simulink model "rx_20140509"  (R2012b)
settings: Solver=ode45  StartTime=0.0  StopTime=10000.0  RelTol=1e-3
libraries: xbsIndex_r4 x2065, casper_library_misc x67, xps_library x56, xbsReplacements_r4 x12, gavrt_library x3, casper_library_sources x2, simulink x1, casper_library_delays x1
(part 1 of 22)
settings Model: Creator=griffin  LastModifiedBy=wnew
settings DataIOCC: SignalLoggingSaveFormat=ModelDataLogs
settings DebuggingCC: FcnCallInpInsideContextMsg=UseLocalSettings  StrictBusMsg=Warning
settings GRTTargetCC: CombineOutputUpdateFcns=off  GRTInterface=on

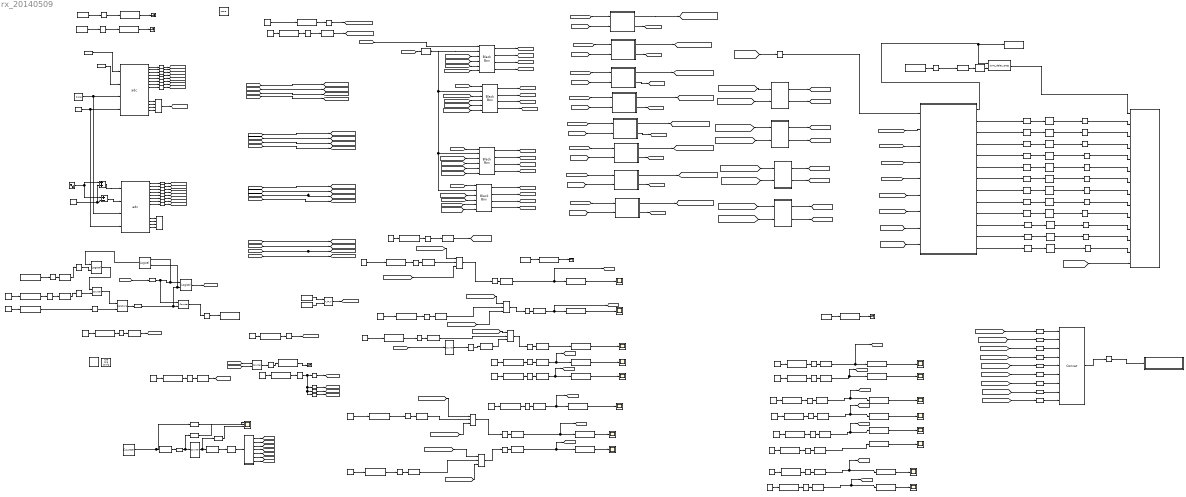
== system rx_20140509 ==
  note: fft_shift: bits 0-15
      | sync_rst: bit 16 -NA
      | arm_rst: bit 17 -NA
      | input_sel: bits 20-22
  note: The FFT Channels are assumed to be
      | Channel1= LCP +TREF (ADC0 I)
      | Channel2=LCP-TREF (ADC0 Q)
      | Channel3=RCP+TREF (ADC1 I)
      | Channel4=RCP-TREF (ADC1 Q)
  note: this shouild sync up the accumulation correctly
  note: To move DC bin higher:
      | Reduce Latency of Sync or increase latency of Data
      | To move DC bin lower:
      | Increase latency of Sync or decrease latency of Data
  note: 0 means Total Power/1 means Poalrimeter
  note: polarimeter versioning begins at 1
  " System Generator" : xbsIndex_r4/ System Generator  Tag=genX  xilinxfamily=virtex5  part=xc5vsx95t  speed=-1  package=ff1136  synthesis_tool=XST  clock_wrapper=Clock Enables  directory=./rx_20140505/sysgen  proj_type=Project Navigator  Synth_file=XST Defaults  Impl_file=ISE Defaults  testbench=off  simulink_period=1  sysclk_period=4  dcm_input_clock_period=100  incr_netlist=off  trim_vbits=Everywhere in SubSystem  dbl_ovrd=According to Block Masks  core_generation=According to Block Masks  run_coregen=off  deprecated_control=off  eval_field=0  block_type=sysgen
      settings: block_version=11.4
  Add2 : Sum
  Add3 : Sum  Inputs=+-
  Band-Limited White Noise1 : simulink/Sources/Band-Limited White Noise  Cov=0.000001  Ts=0.25  seed=[23341]
  Black Box{1..4} (4 alike) : xbsIndex_r4/Black Box  init_code=pfb_blackbox_200mhz_config  sim_method=Inactive  verbose=off  block_type=blackbox2
  Concat : xbsIndex_r4/Concat  num_inputs=9  dbl_ovrd=off  block_type=concat
  Constant{1,3..4,8} (4 alike) : Constant
  Constant{7,9..14,17..21,23..27} (17 alike) : Constant  Value=0
  Constant{2,5,15..16,22} (5 alike) : Constant  Value=30
  Convert : xbsIndex_r4/Convert  gui_display_data_type=Fixed-point  arith_type="Signed  (2's comp)"  n_bits=32  bin_pt=0  float_type=Single  exp_bits=8  fraction_bits=24  quantization=Truncate  overflow=Wrap  en=off  latency=0  dbl_ovrd=off  pipeline=off  block_type=convert
      settings: block_version=11.4
  Convert2 : xbsIndex_r4/Convert  gui_display_data_type=Fixed-point  arith_type=Boolean  n_bits=16  bin_pt=14  float_type=Single  exp_bits=8  fraction_bits=24  quantization=Truncate  overflow=Wrap  en=off  latency=0  dbl_ovrd=off  pipeline=off  block_type=convert
      settings: block_version=11.4
  Counter1 : xbsIndex_r4/Counter  cnt_type=Free Running  cnt_to=Inf  operation=Up  start_count=0  cnt_by_val=1  arith_type=Unsigned  n_bits=10  bin_pt=0  load_pin=off  rst=off  en=off  explicit_period=on  period=1  dbl_ovrd=off  use_behavioral_HDL=off  implementation=Fabric  block_type=counter
      settings: block_version=11.4
  Counter2 : xbsIndex_r4/Counter  cnt_type=Free Running  cnt_to=Inf  operation=Up  start_count=0  cnt_by_val=1  arith_type=Unsigned  n_bits=1  bin_pt=0  load_pin=off  rst=off  en=on  explicit_period=on  period=1  dbl_ovrd=off  use_behavioral_HDL=off  implementation=Fabric  block_type=counter
      settings: block_version=11.4
  Counter3 : xbsIndex_r4/Counter  cnt_type=Free Running  cnt_to=Inf  operation=Up  start_count=0  cnt_by_val=1  arith_type=Unsigned  n_bits=1  bin_pt=0  load_pin=off  rst=off  en=on  explicit_period=on  period=1  dbl_ovrd=off  use_behavioral_HDL=off  implementation=Fabric  block_type=counter
      settings: block_version=11.4
  Delay{,1,3,6,11..18,22,24..31,74..75,83,91} (25 alike) : xbsIndex_r4/Delay  rst=off  infoeditControl=Selection of Reset will increase slice count due to use of real FFs and instead of SRLs  en=off  latency=1  dbl_ovrd=off  reg_retiming=off  block_type=delay
      Delay11 settings: block_version=11.4
      Delay12 settings: block_version=11.4
      Delay13 settings: block_version=11.4
      Delay14 settings: block_version=11.4
      Delay15 settings: block_version=11.4
      Delay16 settings: block_version=11.4
      Delay17 settings: block_version=11.4
      Delay18 settings: block_version=11.4
      Delay22 settings: block_version=11.4
      Delay24 settings: block_version=11.4
      Delay25 settings: block_version=11.4
      Delay26 settings: block_version=11.4
      Delay27 settings: block_version=11.4
      Delay28 settings: block_version=11.4
      Delay29 settings: block_version=11.4
      Delay30 settings: block_version=11.4
  Delay{2,4..5,7..10,19..21,23,32..50,52,54..55,57..58,60,62,65,68,70,73,76..82,84..90,93..102} (65 alike) : xbsIndex_r4/Delay  rst=off  infoeditControl=Selection of Reset will increase slice count due to use of real FFs and instead of SRLs  en=off  latency=2  dbl_ovrd=off  reg_retiming=off  block_type=delay
  Delay{51,53,56,59,61,63..64,66..67,69,71..72} (12 alike) : xbsIndex_r4/Delay  rst=off  infoeditControl=Selection of Reset will increase slice count due to use of real FFs and instead of SRLs  en=off  latency=1  dbl_ovrd=off  reg_retiming=on  block_type=delay
  GPIOA_DIRECTION : xps_library/gpio  Tag=xps:gpio  io_group=ROACH:gpioa_oe_n  io_dir=out  arith_type=Boolean  bitwidth=1  bin_pt=0  bit_index=0  sample_period=1  use_single_ended=off  use_ddr=off  reg_iob=on  reg_clk_phase=0  termination=None
  GPIOB_DIRECTION : xps_library/gpio  Tag=xps:gpio  io_group=ROACH:gpiob_oe_n  io_dir=out  arith_type=Boolean  bitwidth=1  bin_pt=0  bit_index=0  sample_period=1  use_single_ended=off  use_ddr=off  reg_iob=on  reg_clk_phase=0  termination=None
  Imag : xbsIndex_r4/Constant  const=0  gui_display_data_type=Fixed-point  arith_type=Signed (2's comp)  n_bits=18  bin_pt=0  preci_type=Single  exp_width=8  frac_width=24  explicit_period=on  period=1  equ=P=C  opselect=C  inp2=PCIN>>17  opr=+  inp1=P  carry=CIN  dbl_ovrd=off  block_type=constant
      settings: block_version=11.4
  Logical : xbsIndex_r4/Logical  logical_function=OR  inputs=2  en=off  latency=2  precision=Full  arith_type=Unsigned  n_bits=16  bin_pt=0  align_bp=on  dbl_ovrd=off  block_type=logical
      settings: block_version=11.4
  Logical1 : xbsIndex_r4/Logical  logical_function=OR  inputs=4  en=off  latency=1  precision=Full  arith_type=Unsigned  n_bits=8  bin_pt=2  align_bp=on  dbl_ovrd=off  block_type=logical
      settings: xl_area=[1 1 0 1 0 0 0]
  Logical2 : xbsIndex_r4/Logical  logical_function=OR  inputs=2  en=off  latency=2  precision=Full  arith_type=Unsigned  n_bits=16  bin_pt=0  align_bp=on  dbl_ovrd=off  block_type=logical
      settings: block_version=11.4
  Logical3 : xbsIndex_r4/Logical  logical_function=OR  inputs=4  en=off  latency=1  precision=Full  arith_type=Unsigned  n_bits=8  bin_pt=2  align_bp=on  dbl_ovrd=off  block_type=logical
      settings: xl_area=[1 1 0 1 0 0 0]
  Logical4 : xbsIndex_r4/Logical  logical_function=OR  inputs=2  en=off  latency=2  precision=Full  arith_type=Unsigned  n_bits=16  bin_pt=0  align_bp=on  dbl_ovrd=off  block_type=logical
      settings: block_version=11.4
  Mux{,1..4} (5 alike) : xbsIndex_r4/Mux  inputs=2  en=off  latency=0  precision=Full  arith_type=Unsigned  n_bits=16  bin_pt=14  quantization=Truncate  overflow=Wrap  dbl_ovrd=off  block_type=mux
      settings: block_version=11.4
  Pulse Generator : DiscretePulseGenerator  Period=2^27
  Real : xbsIndex_r4/Constant  const=1  gui_display_data_type=Fixed-point  arith_type=Signed (2's comp)  n_bits=18  bin_pt=0  preci_type=Single  exp_width=8  frac_width=24  explicit_period=on  period=1  equ=P=C  opselect=C  inp2=PCIN>>17  opr=+  inp1=P  carry=CIN  dbl_ovrd=off  block_type=constant
      settings: block_version=11.4
  Real1 : xbsIndex_r4/Constant  const=0  gui_display_data_type=Fixed-point  arith_type=Boolean  n_bits=18  bin_pt=0  preci_type=Single  exp_width=8  frac_width=24  explicit_period=on  period=1  equ=P=C  opselect=C  inp2=PCIN>>17  opr=+  inp1=P  carry=CIN  dbl_ovrd=off  block_type=constant
      settings: block_version=11.4
  Real2 : xbsIndex_r4/Constant  const=0  gui_display_data_type=Fixed-point  arith_type=Boolean  n_bits=18  bin_pt=0  preci_type=Single  exp_width=8  frac_width=24  explicit_period=on  period=1  equ=P=C  opselect=C  inp2=PCIN>>17  opr=+  inp1=P  carry=CIN  dbl_ovrd=off  block_type=constant
      settings: block_version=11.4
  Real6 : xbsIndex_r4/Constant  const=1  gui_display_data_type=Fixed-point  arith_type=Unsigned  n_bits=18  bin_pt=0  preci_type=Single  exp_width=8  frac_width=24  explicit_period=on  period=1  equ=P=C  opselect=C  inp2=PCIN>>17  opr=+  inp1=P  carry=CIN  dbl_ovrd=off  block_type=constant
      settings: block_version=11.4
  Real7 : xbsIndex_r4/Constant  const=1  gui_display_data_type=Fixed-point  arith_type=Unsigned  n_bits=18  bin_pt=0  preci_type=Single  exp_width=8  frac_width=24  explicit_period=on  period=1  equ=P=C  opselect=C  inp2=PCIN>>17  opr=+  inp1=P  carry=CIN  dbl_ovrd=off  block_type=constant
      settings: block_version=11.4
  Reinterpret : xbsIndex_r4/Reinterpret  force_arith_type=on  arith_type=Unsigned  force_bin_pt=on  bin_pt=0  block_type=reinterpret
      settings: infoedit="Changes signal type without altering the binary representation.   You can changed the signal between signed and unsigned, and relocate the binary point.<br><br>Hardware notes: In hardware this block costs nothing.<br><br>Example:  Suppose the input is 6 bits wide, signed, with 2 fractional bits, and the output is forced to unsigned with 0 fractional bits.  Then an input of -2.0 (1110.00 in binary 2's complement) becomes an output of 56 (111000 in binary)."
  Relational : xbsIndex_r4/Relational  mode=a>b  en=off  latency=2  dbl_ovrd=off  block_type=relational
  Scope{,1..3,5..16} (16 alike) : Scope
      Scope settings: SaveName=ScopeData4
      Scope1 settings: SaveName=ScopeData10
      Scope10 settings: SaveName=ScopeData2
      Scope11 settings: YMin=0  YMax=1  SaveName=ScopeData3
      Scope12 settings: SaveName=ScopeData13
      Scope13 settings: SaveName=ScopeData14
      Scope14 settings: SaveName=ScopeData15
      Scope15 settings: SaveName=ScopeData16
      Scope16 settings: SaveName=ScopeData17
      Scope2 settings: YMin=0  YMax=1  SaveName=ScopeData11
      Scope5 settings: SaveName=ScopeData12
      Scope6 settings: SaveName=ScopeData7
      Scope7 settings: SaveName=ScopeData8
      Scope8 settings: SaveName=ScopeData9
      Scope9 settings: SaveName=ScopeData18
  Scope4 : Scope  NumInputPorts=3
      settings: YMin=-5~-5~-5  YMax=5~5~5
  Sine Wave1 : Sin  Amplitude=0.00001  Frequency=5  Phase=1.57  SampleTime=0.25
  Slice1 : xbsIndex_r4/Slice  nbits=1  boolean_output=on  mode=Upper Bit Location + Width  bit1=0  base1=LSB of Input  bit0=0  base0=LSB of Input  dbl_ovrd=off  block_type=slice
  Slice{5,9..17,21,23..36} (25 alike) : xbsIndex_r4/Slice  nbits=1  boolean_output=on  mode=Lower Bit Location + Width  bit1=0  base1=LSB of Input  bit0=0  base0=LSB of Input  dbl_ovrd=off  block_type=slice
  Slice18 : xbsIndex_r4/Slice  nbits=16  boolean_output=off  mode=Lower Bit Location + Width  bit1=0  base1=MSB of Input  bit0=0  base0=LSB of Input  dbl_ovrd=off  block_type=slice
      settings: infoedit="Extracts a given range of bits from each input sample and presents it at the output.  The output type is ordinarily unsigned with binary point at zero, but can be Boolean when the slice is one bit wide.<P><P>Hardware notes: In hardware this block costs nothing."  block_version=10.1.3
  Slice19 : xbsIndex_r4/Slice  nbits=1  boolean_output=on  mode=Lower Bit Location + Width  bit1=0  base1=MSB of Input  bit0=16  base0=LSB of Input  dbl_ovrd=off  block_type=slice
      settings: infoedit="Extracts a given range of bits from each input sample and presents it at the output.  The output type is ordinarily unsigned with binary point at zero, but can be Boolean when the slice is one bit wide.<P><P>Hardware notes: In hardware this block costs nothing."  block_version=10.1.3
  Slice2 : xbsIndex_r4/Slice  nbits=1  boolean_output=on  mode=Upper Bit Location + Width  bit1=0  base1=LSB of Input  bit0=0  base0=LSB of Input  dbl_ovrd=off  block_type=slice
  Slice20 : xbsIndex_r4/Slice  nbits=6  boolean_output=off  mode=Lower Bit Location + Width  bit1=0  base1=LSB of Input  bit0=0  base0=LSB of Input  dbl_ovrd=off  block_type=slice
  Slice22 : xbsIndex_r4/Slice  nbits=1  boolean_output=on  mode=Lower Bit Location + Width  bit1=0  base1=MSB of Input  bit0=17  base0=LSB of Input  dbl_ovrd=off  block_type=slice
      settings: infoedit="Extracts a given range of bits from each input sample and presents it at the output.  The output type is ordinarily unsigned with binary point at zero, but can be Boolean when the slice is one bit wide.<P><P>Hardware notes: In hardware this block costs nothing."  block_version=10.1.3
  Slice3 : xbsIndex_r4/Slice  nbits=3  boolean_output=off  mode=Lower Bit Location + Width  bit1=0  base1=MSB of Input  bit0=20  base0=LSB of Input  dbl_ovrd=off  block_type=slice
      settings: infoedit="Extracts a given range of bits from each input sample and presents it at the output.  The output type is ordinarily unsigned with binary point at zero, but can be Boolean when the slice is one bit wide.<P><P>Hardware notes: In hardware this block costs nothing."  block_version=10.1.3
  Slice4 : xbsIndex_r4/Slice  nbits=1  boolean_output=on  mode=Upper Bit Location + Width  bit1=0  base1=MSB of Input  bit0=0  base0=LSB of Input  dbl_ovrd=off  block_type=slice
  Slice7 : xbsIndex_r4/Slice  nbits=1  boolean_output=on  mode=Lower Bit Location + Width  bit1=-1  base1=MSB of Input  bit0=0  base0=LSB of Input  dbl_ovrd=off  block_type=slice
  Slice8 : xbsIndex_r4/Slice  nbits=1  boolean_output=on  mode=Lower Bit Location + Width  bit1=-1  base1=MSB of Input  bit0=0  base0=LSB of Input  dbl_ovrd=off  block_type=slice
  StokesDetector : Subsystem  AncestorBlock=gavrt_library/StokesDetector  mask(stokes){bit_width=18, add_latency=2, mult_latency=3}
      mask prompts: bit_width "Bit Width"; add_latency "Add Latency"; mult_latency "Mult Latency"
      mask help: Compute cross products necessary for full stokes parameters
  Subsystem1 : Subsystem
  Subsystem2 : Subsystem
  Subsystem3 : Subsystem
  Subsystem4 : Subsystem
  Subsystem5 : Subsystem
  Terminator{,1..4} (5 alike) : Terminator
  Walshing1 : Subsystem
  XSG core config : xps_library/XSG core config  Tag=xps:xsg  hw_sys=ROACH:sx95t  clk_src=adc0_clk  ROACH_clk_src=adc0_clk  ROACH2_clk_src=adc0_clk  clk_rate=250  sample_period=1  synthesis_tool=XST
  acc_len : xps_library/software register  Tag=xps:sw_reg  io_dir=From Processor  arith_type=Unsigned  bitwidth=32  bin_pt=0  sample_period=1  gw_name=rx_20140509_acc_len_user_data_out
  acc_sync_delay : xps_library/software register  Tag=xps:sw_reg  io_dir=From Processor  arith_type=Unsigned  bitwidth=32  bin_pt=0  sample_period=1  gw_name=rx_20140509_acc_sync_delay_user_data_out
  adc0 : xps_library/adc  Tag=xps:adc  adc_brd=adc0  adc_clk_rate=1000  adc_interleave=off  sample_period=1
  adc1 : xps_library/adc  Tag=xps:adc  adc_brd=adc1  adc_clk_rate=1000  adc_interleave=off  sample_period=1
  amp_EQ0 : Subsystem  mask{N=5, bram_lat=2, mult_lat=3, add_lat=2}
      mask prompts: N "number of coefficients (2^?)"; bram_lat "bram latency"; mult_lat "multiplier latency"; add_lat "adder latency"
  amp_EQ1 : Subsystem  mask{N=5, bram_lat=2, mult_lat=3, add_lat=2}
      mask prompts: N "number of coefficients (2^?)"; bram_lat "bram latency"; mult_lat "multiplier latency"; add_lat "adder latency"
  amp_EQ2 : Subsystem  mask{N=5, bram_lat=2, mult_lat=3, add_lat=2}
      mask prompts: N "number of coefficients (2^?)"; bram_lat "bram latency"; mult_lat "multiplier latency"; add_lat "adder latency"
  amp_EQ3 : Subsystem  mask{N=5, bram_lat=2, mult_lat=3, add_lat=2}
      mask prompts: N "number of coefficients (2^?)"; bram_lat "bram latency"; mult_lat "multiplier latency"; add_lat "adder latency"
  amp_EQ4 : Subsystem  mask{N=5, bram_lat=2, mult_lat=3, add_lat=2}
      mask prompts: N "number of coefficients (2^?)"; bram_lat "bram latency"; mult_lat "multiplier latency"; add_lat "adder latency"
  amp_EQ5 : Subsystem  mask{N=5, bram_lat=2, mult_lat=3, add_lat=2}
      mask prompts: N "number of coefficients (2^?)"; bram_lat "bram latency"; mult_lat "multiplier latency"; add_lat "adder latency"
  amp_EQ6 : Subsystem  mask{N=5, bram_lat=2, mult_lat=3, add_lat=2}
      mask prompts: N "number of coefficients (2^?)"; bram_lat "bram latency"; mult_lat "multiplier latency"; add_lat "adder latency"
  amp_EQ7 : Subsystem  mask{N=5, bram_lat=2, mult_lat=3, add_lat=2}
      mask prompts: N "number of coefficients (2^?)"; bram_lat "bram latency"; mult_lat "multiplier latency"; add_lat "adder latency"
  bofMode : xps_library/software register  Tag=xps:sw_reg  io_dir=From Processor  arith_type=Unsigned  bitwidth=32  bin_pt=0  sample_period=1  gw_name=rx_20140509_bofMode_user_data_out
  bofVersion : xps_library/software register  Tag=xps:sw_reg  io_dir=From Processor  arith_type=Unsigned  bitwidth=32  bin_pt=0  sample_period=1  gw_name=rx_20140509_bofVersion_user_data_out
  cnt_rst : xps_library/software register  Tag=xps:sw_reg  io_dir=From Processor  arith_type=Unsigned  bitwidth=32  bin_pt=0  sample_period=1  gw_name=rx_20140509_cnt_rst_user_data_out
  ctrl_sw : xps_library/software register  Tag=xps:sw_reg  io_dir=From Processor  arith_type=Unsigned  bitwidth=32  bin_pt=0  sample_period=1  gw_name=rx_20140509_ctrl_sw_user_data_out
  demodPhaseSwitch1 : xps_library/software register  Tag=xps:sw_reg  io_dir=From Processor  arith_type=Unsigned  bitwidth=32  bin_pt=0  sample_period=1  gw_name=rx_20140509_demodPhaseSwitch1_user_data_out
  gpio : xps_library/gpio  Tag=xps:gpio  io_group=ROACH:gpioa  io_dir=out  arith_type=Boolean  bitwidth=1  bin_pt=0  bit_index=0  sample_period=1  use_single_ended=off  use_ddr=off  reg_iob=on  reg_clk_phase=0  termination=None
  gpio1 : xps_library/gpio  Tag=xps:gpio  io_group=ROACH:gpioa  io_dir=out  arith_type=Boolean  bitwidth=1  bin_pt=0  bit_index=1  sample_period=1  use_single_ended=off  use_ddr=off  reg_iob=on  reg_clk_phase=0  termination=None
  gpio10 : xps_library/gpio  Tag=xps:gpio  io_group=ROACH:gpiob  io_dir=out  arith_type=Boolean  bitwidth=1  bin_pt=0  bit_index=2  sample_period=1  use_single_ended=off  use_ddr=off  reg_iob=on  reg_clk_phase=0  termination=None
  gpio11 : xps_library/gpio  Tag=xps:gpio  io_group=ROACH:gpiob  io_dir=out  arith_type=Boolean  bitwidth=1  bin_pt=0  bit_index=3  sample_period=1  use_single_ended=off  use_ddr=off  reg_iob=on  reg_clk_phase=0  termination=None
  gpio12 : xps_library/gpio  Tag=xps:gpio  io_group=ROACH:gpiob  io_dir=out  arith_type=Boolean  bitwidth=1  bin_pt=0  bit_index=4  sample_period=1  use_single_ended=off  use_ddr=off  reg_iob=on  reg_clk_phase=0  termination=None
  gpio13 : xps_library/gpio  Tag=xps:gpio  io_group=ROACH:gpiob  io_dir=out  arith_type=Boolean  bitwidth=1  bin_pt=0  bit_index=5  sample_period=1  use_single_ended=off  use_ddr=off  reg_iob=on  reg_clk_phase=0  termination=None
  gpio14 : xps_library/gpio  Tag=xps:gpio  io_group=ROACH:gpiob  io_dir=out  arith_type=Boolean  bitwidth=1  bin_pt=0  bit_index=6  sample_period=1  use_single_ended=off  use_ddr=off  reg_iob=on  reg_clk_phase=0  termination=None
  gpio15 : xps_library/gpio  Tag=xps:gpio  io_group=ROACH:gpiob  io_dir=out  arith_type=Boolean  bitwidth=1  bin_pt=0  bit_index=7  sample_period=1  use_single_ended=off  use_ddr=off  reg_iob=on  reg_clk_phase=0  termination=None
  gpio2 : xps_library/gpio  Tag=xps:gpio  io_group=ROACH:gpioa  io_dir=out  arith_type=Boolean  bitwidth=1  bin_pt=0  bit_index=2  sample_period=1  use_single_ended=off  use_ddr=off  reg_iob=on  reg_clk_phase=0  termination=None
  gpio3 : xps_library/gpio  Tag=xps:gpio  io_group=ROACH:gpioa  io_dir=out  arith_type=Boolean  bitwidth=1  bin_pt=0  bit_index=3  sample_period=1  use_single_ended=off  use_ddr=off  reg_iob=on  reg_clk_phase=0  termination=None
  gpio4 : xps_library/gpio  Tag=xps:gpio  io_group=ROACH:gpioa  io_dir=out  arith_type=Boolean  bitwidth=1  bin_pt=0  bit_index=4  sample_period=1  use_single_ended=off  use_ddr=off  reg_iob=on  reg_clk_phase=0  termination=None
  gpio5 : xps_library/gpio  Tag=xps:gpio  io_group=ROACH:gpioa  io_dir=out  arith_type=Boolean  bitwidth=1  bin_pt=0  bit_index=5  sample_period=1  use_single_ended=off  use_ddr=off  reg_iob=on  reg_clk_phase=0  termination=None
  gpio6 : xps_library/gpio  Tag=xps:gpio  io_group=ROACH:gpioa  io_dir=out  arith_type=Boolean  bitwidth=1  bin_pt=0  bit_index=6  sample_period=1  use_single_ended=off  use_ddr=off  reg_iob=on  reg_clk_phase=0  termination=None
  gpio7 : xps_library/gpio  Tag=xps:gpio  io_group=ROACH:gpioa  io_dir=out  arith_type=Boolean  bitwidth=1  bin_pt=0  bit_index=7  sample_period=1  use_single_ended=off  use_ddr=off  reg_iob=on  reg_clk_phase=0  termination=None
  gpio8 : xps_library/gpio  Tag=xps:gpio  io_group=ROACH:gpiob  io_dir=out  arith_type=Boolean  bitwidth=1  bin_pt=0  bit_index=0  sample_period=1  use_single_ended=off  use_ddr=off  reg_iob=on  reg_clk_phase=0  termination=None
  gpio9 : xps_library/gpio  Tag=xps:gpio  io_group=ROACH:gpiob  io_dir=out  arith_type=Boolean  bitwidth=1  bin_pt=0  bit_index=1  sample_period=1  use_single_ended=off  use_ddr=off  reg_iob=on  reg_clk_phase=0  termination=None
  gpioMode : xps_library/software register  Tag=xps:sw_reg  io_dir=From Processor  arith_type=Unsigned  bitwidth=32  bin_pt=0  sample_period=1  gw_name=rx_20140509_gpioMode_user_data_out
  gpio_set0 : xps_library/software register  Tag=xps:sw_reg  io_dir=From Processor  arith_type=Unsigned  bitwidth=32  bin_pt=0  sample_period=1  gw_name=rx_20140509_gpio_set0_user_data_out
  gpio_set1 : xps_library/software register  Tag=xps:sw_reg  io_dir=From Processor  arith_type=Unsigned  bitwidth=32  bin_pt=0  sample_period=1  gw_name=rx_20140509_gpio_set1_user_data_out
  gpio_set2 : xps_library/software register  Tag=xps:sw_reg  io_dir=From Processor  arith_type=Unsigned  bitwidth=32  bin_pt=0  sample_period=1  gw_name=rx_20140509_gpio_set2_user_data_out
  gpio_set3 : xps_library/software register  Tag=xps:sw_reg  io_dir=From Processor  arith_type=Unsigned  bitwidth=32  bin_pt=0  sample_period=1  gw_name=rx_20140509_gpio_set3_user_data_out
  gpio_set4 : xps_library/software register  Tag=xps:sw_reg  io_dir=From Processor  arith_type=Unsigned  bitwidth=32  bin_pt=0  sample_period=1  gw_name=rx_20140509_gpio_set4_user_data_out
  gpio_set5 : xps_library/software register  Tag=xps:sw_reg  io_dir=From Processor  arith_type=Unsigned  bitwidth=32  bin_pt=0  sample_period=1  gw_name=rx_20140509_gpio_set5_user_data_out
  gpio_set6 : xps_library/software register  Tag=xps:sw_reg  io_dir=From Processor  arith_type=Unsigned  bitwidth=32  bin_pt=0  sample_period=1  gw_name=rx_20140509_gpio_set6_user_data_out
  gpio_set7 : xps_library/software register  Tag=xps:sw_reg  io_dir=From Processor  arith_type=Unsigned  bitwidth=32  bin_pt=0  sample_period=1  gw_name=rx_20140509_gpio_set7_user_data_out
  gpiob_set0 : xps_library/software register  Tag=xps:sw_reg  io_dir=From Processor  arith_type=Unsigned  bitwidth=32  bin_pt=0  sample_period=1  gw_name=rx_20140509_gpiob_set0_user_data_out
  gpiob_set1 : xps_library/software register  Tag=xps:sw_reg  io_dir=From Processor  arith_type=Unsigned  bitwidth=32  bin_pt=0  sample_period=1  gw_name=rx_20140509_gpiob_set1_user_data_out
  gpiob_set2 : xps_library/software register  Tag=xps:sw_reg  io_dir=From Processor  arith_type=Unsigned  bitwidth=32  bin_pt=0  sample_period=1  gw_name=rx_20140509_gpiob_set2_user_data_out
  gpiob_set3 : xps_library/software register  Tag=xps:sw_reg  io_dir=From Processor  arith_type=Unsigned  bitwidth=32  bin_pt=0  sample_period=1  gw_name=rx_20140509_gpiob_set3_user_data_out
  gpiob_set4 : xps_library/software register  Tag=xps:sw_reg  io_dir=From Processor  arith_type=Unsigned  bitwidth=32  bin_pt=0  sample_period=1  gw_name=rx_20140509_gpiob_set4_user_data_out
  gpiob_set5 : xps_library/software register  Tag=xps:sw_reg  io_dir=From Processor  arith_type=Unsigned  bitwidth=32  bin_pt=0  sample_period=1  gw_name=rx_20140509_gpiob_set5_user_data_out
  gpiob_set6 : xps_library/software register  Tag=xps:sw_reg  io_dir=From Processor  arith_type=Unsigned  bitwidth=32  bin_pt=0  sample_period=1  gw_name=rx_20140509_gpiob_set6_user_data_out
  gpiob_set7 : xps_library/software register  Tag=xps:sw_reg  io_dir=From Processor  arith_type=Unsigned  bitwidth=32  bin_pt=0  sample_period=1  gw_name=rx_20140509_gpiob_set7_user_data_out
  no_PPS_cnt : xps_library/software register  Tag=xps:sw_reg  io_dir=To Processor  arith_type=Unsigned  bitwidth=32  bin_pt=0  sample_period=1  gw_name=rx_20140509_no_PPS_cnt_user_data_in
  out : xbsIndex_r4/Gateway Out  inherit_from_input=off  hdl_port=on  timing_constraint=None  locs_specified=off  LOCs={}  UseAsDAC=off  DACChannel='1'  block_type=gatewayout
      settings: infoedit="Gateway out block.  Converts Xilinx fixed point inputs into ouputs of type Simulink integer, double, or fixed point.<br><br>Hardware notes:  In hardware these blocks become top level output ports or are discarded, depending on how they are configured."  block_version=11.4
  out1 : xbsIndex_r4/Gateway Out  inherit_from_input=off  hdl_port=on  timing_constraint=None  locs_specified=off  LOCs={}  UseAsDAC=off  DACChannel='1'  block_type=gatewayout
      settings: infoedit="Gateway out block.  Converts Xilinx fixed point inputs into ouputs of type Simulink integer, double, or fixed point.<br><br>Hardware notes:  In hardware these blocks become top level output ports or are discarded, depending on how they are configured."  block_version=11.4
  out2 : xbsIndex_r4/Gateway Out  inherit_from_input=off  hdl_port=on  timing_constraint=None  locs_specified=off  LOCs={}  UseAsDAC=off  DACChannel='1'  block_type=gatewayout
      settings: infoedit="Gateway out block.  Converts Xilinx fixed point inputs into ouputs of type Simulink integer, double, or fixed point.<br><br>Hardware notes:  In hardware these blocks become top level output ports or are discarded, depending on how they are configured."  block_version=11.4
  pcore : xps_library/pcore  Tag=xps:pcore  pcore_path=./pfb_blackbox_200mhz_core/pfb_blackbox_200mhz.ngc
  phaseDelay2 : xps_library/software register  Tag=xps:sw_reg  io_dir=From Processor  arith_type=Unsigned  bitwidth=32  bin_pt=0  sample_period=1  gw_name=rx_20140509_phaseDelay2_user_data_out
  posedge1 : casper_library_misc/posedge  Tag=Rising Edge Detector
  posedge2 : casper_library_misc/posedge  Tag=Rising Edge Detector
  posedge6 : casper_library_misc/posedge  Tag=Rising Edge Detector
  pure_tone_gen : casper_library_sources/pure_tone_gen  adc_demux_factor=8  num_fft_channels=32  tone_channel=10
  pure_tone_gen1 : casper_library_sources/pure_tone_gen  adc_demux_factor=8  num_fft_channels=32  tone_channel=10
  ri_to_c8 : casper_library_misc/ri_to_c
  snap_we : xps_library/software register  Tag=xps:sw_reg  io_dir=From Processor  arith_type=Unsigned  bitwidth=32  bin_pt=0  sample_period=1  gw_name=rx_20140509_snap_we_user_data_out
  statusReadout : Subsystem  Tag=xps:sw_reg  mask{io_dir=To Processor, arith_type=Unsigned, bitwidth=32, bin_pt=0, sample_period=1, latency=0}
      mask prompts: io_dir "I/O direction"; arith_type "Data Type"; bitwidth "Data bitwidth"; bin_pt "Data binary point"; sample_period "Sample period"
      mask init:
      | gw_name = clear_name(gcb);
      | config.source = str2func('software_register_init');
      | config.toplevel = gcb;
      | xBlock( config, {io_dir, arith_type, bitwidth, bin_pt, ... 
      |     sample_period, gw_name, latency});
      mask TypeOptions io_dir: From Processor | To Processor
      mask TypeOptions arith_type: Unsigned | Signed  (2's comp)
  sync : xbsIndex_r4/Counter  cnt_type=Free Running  cnt_to=Inf  operation=Up  start_count=0  cnt_by_val=1  arith_type=Unsigned  n_bits=29  bin_pt=0  load_pin=off  rst=on  en=on  explicit_period=on  period=1  dbl_ovrd=off  use_behavioral_HDL=off  implementation=Fabric  block_type=counter
      settings: block_version=11.4
  sync1 : xbsIndex_r4/Counter  cnt_type=Free Running  cnt_to=Inf  operation=Up  start_count=0  cnt_by_val=1  arith_type=Unsigned  n_bits=29  bin_pt=0  load_pin=off  rst=on  en=on  explicit_period=on  period=1  dbl_ovrd=off  use_behavioral_HDL=off  implementation=Fabric  block_type=counter
      settings: block_version=11.4
  sync_cnt : xps_library/software register  Tag=xps:sw_reg  io_dir=To Processor  arith_type=Unsigned  bitwidth=32  bin_pt=0  sample_period=1  gw_name=rx_20140509_sync_cnt_user_data_in
  sync_cnt1 : xps_library/software register  Tag=xps:sw_reg  io_dir=To Processor  arith_type=Unsigned  bitwidth=32  bin_pt=0  sample_period=1  gw_name=rx_20140509_sync_cnt1_user_data_in
  sync_cntr : xbsIndex_r4/Counter  cnt_type=Free Running  cnt_to=Inf  operation=Up  start_count=0  cnt_by_val=1  arith_type=Unsigned  n_bits=32  bin_pt=0  load_pin=off  rst=on  en=on  explicit_period=on  period=1  dbl_ovrd=off  use_behavioral_HDL=off  implementation=Fabric  block_type=counter
      settings: block_version=11.4
  sync_delay_prog : casper_library_delays/sync_delay_prog  MaxDelay=6
  sync_en : xps_library/software register  Tag=xps:sw_reg  io_dir=From Processor  arith_type=Unsigned  bitwidth=32  bin_pt=0  sample_period=1  gw_name=rx_20140509_sync_en_user_data_out
  sync_max : xps_library/software register  Tag=xps:sw_reg  io_dir=From Processor  arith_type=Unsigned  bitwidth=32  bin_pt=0  sample_period=1  gw_name=rx_20140509_sync_max_user_data_out
  sync_rst : xps_library/software register  Tag=xps:sw_reg  io_dir=From Processor  arith_type=Unsigned  bitwidth=32  bin_pt=0  sample_period=1  gw_name=rx_20140509_sync_rst_user_data_out
      link override rx_25May_stat_sync_rst_user_data_out: gui_display_data_type=Boolean  arith_type=Boolean  n_bits=32  bin_pt=0  preci_type=Single  exp_width=8  frac_width=24  quantization="Round  (unbiased: +/- Inf)"  overflow=Saturate  period=1  dbl_ovrd=off  timing_constraint=None  locs_specified=off  LOCs={}  UseAsADC=off  ADCChannel='1'  inherit_from_input=off  hdl_port=on
      link override rx_25May_stat_sync_rst_user_data_out: infoedit="Gateway in block.  Converts inputs of type Simulink integer, single, double and fixed-point to  Xilinx fixed-point or floating-point data type.<br><br>Hardware notes:  In hardware these blocks become top level input ports."
  wires:
  Slice22/1 -> [arm_rst]
  Slice19/1 -> [sync_rst]
  Slice18/1 -> [fft_shift]
  Slice3/1 -> [input_sel]
  Delay/1 -> Slice3/1, Slice22/1, Slice19/1, Slice18/1
  ctrl_sw/1 -> Delay/1
  Constant18/1 -> ctrl_sw/1
  Imag/1 -> ri_to_c8/2
  ri_to_c8/1 -> [unity]
  Real/1 -> ri_to_c8/1
  acc_len/1 -> Delay1/1
  Constant2/1 -> acc_len/1
  Delay1/1 -> [acc_len]
  Delay2/1 -> sync_cnt/1
  sync_cntr/1 -> Delay2/1
  sync_cnt/1 -> Terminator/1
  [sync_gen] -> sync_cntr/2
  cnt_rst/1 -> Delay4/1
  Delay4/1 -> Slice1/1
  Slice1/1 -> [cnt_rst]
  Constant3/1 -> cnt_rst/1
  [cnt_rst] -> sync_cntr/1
  Pulse Generator/1 -> adc0/3, adc1/3
  Constant1/1 -> adc0/4, adc1/4
  adc0/13 -> Logical3/1
  adc0/14 -> Logical3/2
  adc0/15 -> Logical3/3
  adc0/16 -> Logical3/4
  adc0/1 -> Delay22/1
  adc0/2 -> Delay24/1
  adc0/3 -> Delay25/1
  adc0/4 -> Delay26/1
  adc0/5 -> Delay27/1
  adc0/6 -> Delay28/1
  adc0/7 -> Delay29/1
  adc0/8 -> Delay30/1
  Logical3/1 -> [sync_adc0]
  Delay22/1 -> [adc0_lcp0]
  Delay24/1 -> [adc0_lcp1]
  Delay25/1 -> [adc0_lcp2]
  Delay26/1 -> [adc0_lcp3]
  Delay27/1 -> [adc0_lcp0a]
  Delay28/1 -> [adc0_lcp1a]
  Delay29/1 -> [adc0_lcp2a]
  Delay30/1 -> [adc0_lcp3a]
  adc1/13 -> Logical1/1
  adc1/14 -> Logical1/2
  adc1/15 -> Logical1/3
  adc1/16 -> Logical1/4
  adc1/1 -> Delay11/1
  adc1/2 -> Delay12/1
  adc1/3 -> Delay13/1
  adc1/4 -> Delay14/1
  adc1/5 -> Delay15/1
  adc1/6 -> Delay16/1
  adc1/7 -> Delay17/1
  adc1/8 -> Delay18/1
  Delay11/1 -> [adc0_rcp0]
  Delay12/1 -> [adc0_rcp1]
  Delay13/1 -> [adc0_rcp2]
  Delay14/1 -> [adc0_rcp3]
  Delay15/1 -> [adc0_rcp0a]
  Delay16/1 -> [adc0_rcp1a]
  Delay17/1 -> [adc0_rcp2a]
  Delay18/1 -> [adc0_rcp3a]
  pure_tone_gen/1 -> adc0/1
  pure_tone_gen1/1 -> adc0/2
  Add2/1 -> adc1/1
  Add3/1 -> adc1/2
  Band-Limited White Noise1/1 -> Add3/2, Add2/2
  Sine Wave1/1 -> Add2/1, Add3/1
  snap_we/1 -> Delay5/1
  Delay5/1 -> Slice2/1
  Slice2/1 -> [snap_we]
  Constant4/1 -> snap_we/1
  [sync_gen] -> Black Box3/1
  [adc0_lcp3demod] -> Black Box3/6
  [adc0_lcp0demod] -> Black Box3/3
  [adc0_lcp1demod] -> Black Box3/4
  [adc0_lcp2demod] -> Black Box3/5
  Black Box3/1 -> [fft0_sync]
  Black Box3/2 -> [fft0_lcp_even]
  Black Box3/3 -> [fft0_lcp_odd]
  Black Box3/4 -> [fft0_of]
  [sync_gen] -> Black Box1/1
  [adc0_lcp0ademod] -> Black Box1/3
  [adc0_lcp1ademod] -> Black Box1/4
  [adc0_lcp2ademod] -> Black Box1/5
  [adc0_lcp3ademod] -> Black Box1/6
  Black Box1/1 -> [fft1_sync]
  Black Box1/2 -> [fft1_lcp_even]
  Black Box1/3 -> [fft1_lcp_odd]
  Black Box1/4 -> [fft1_of]
  [sync_gen] -> Black Box2/1
  [adc0_rcp0ademod] -> Black Box2/3
  [adc0_rcp1ademod] -> Black Box2/4
  [adc0_rcp2ademod] -> Black Box2/5
  [adc0_rcp3ademod] -> Black Box2/6
  [sync_gen] -> Black Box4/1
  [adc0_rcp0demod] -> Black Box4/3
  [adc0_rcp1demod] -> Black Box4/4
  [adc0_rcp2demod] -> Black Box4/5
  [adc0_rcp3demod] -> Black Box4/6
  Black Box4/1 -> [fft2_sync]
  Black Box4/2 -> [fft2_rcp_even]
  Black Box4/3 -> [fft2_rcp_odd]
  Black Box4/4 -> [fft2_of]
  Black Box2/1 -> [fft3_sync]
  Black Box2/2 -> [fft3_rcp_even]
  Black Box2/3 -> [fft3_rcp_odd]
  Black Box2/4 -> [fft3_of]
  [fft_shift] -> Convert/1
  Convert/1 -> Black Box3/2, Black Box1/2, Black Box2/2, Black Box4/2
  Real1/1 -> GPIOA_DIRECTION/1
  GPIOA_DIRECTION/1 -> Terminator3/1
  [fft0_sync] -> amp_EQ1/1(sync_in)
  [fft0_lcp_odd] -> amp_EQ1/2(din)
  [fft0_lcp_even] -> amp_EQ0/2(din)
  [fft0_sync] -> amp_EQ0/1(sync_in)
  [fft1_sync] -> amp_EQ3/1(sync_in)
  [fft1_lcp_odd] -> amp_EQ3/2(din)
  [fft1_sync] -> amp_EQ2/1(sync_in)
  [fft1_lcp_even] -> amp_EQ2/2(din)
  [fft2_sync] -> amp_EQ5/1(sync_in)
  [fft2_rcp_odd] -> amp_EQ5/2(din)
  [fft2_sync] -> amp_EQ4/1(sync_in)
  [fft2_rcp_even] -> amp_EQ4/2(din)
  [fft3_sync] -> amp_EQ7/1(sync_in)
  [fft3_rcp_odd] -> amp_EQ7/2(din)
  [fft3_sync] -> amp_EQ6/1(sync_in)
  [fft3_rcp_even] -> amp_EQ6/2(din)
  Walshing1/1(Out1) -> [wal0]
  Walshing1/2(Out2) -> [wal1]
  Walshing1/3(Out3) -> [wal2]
  Walshing1/4(Out4) -> [wal3]
  Walshing1/5(Out5) -> [wal4]
  Walshing1/6(Out6) -> [wal5]
  Walshing1/7(Out7) -> [wal6]
  Counter1/1 -> out/1, Slice4/1
  Counter3/1 -> Slice10/1, out2/1
  Slice10/1 -> Convert2/1
  Convert2/1 -> Walshing1/1(CLK)
  out/1 -> Scope4/1
  out1/1 -> Scope4/2
  out2/1 -> Scope4/3
  posedge2/1 -> Counter3/1, out1/1
  Slice4/1 -> posedge2/1
  gpio2/1 -> Scope2/1
  Slice9/1 -> gpio2/1
  Delay20/1 -> Slice9/1
  gpio_set3/1 -> Delay19/1
  Constant9/1 -> gpio_set3/1
  gpio3/1 -> Scope3/1
  Slice5/1 -> gpio3/1, [gpioa3]
  Delay19/1 -> Slice5/1
  Delay41/1 -> Slice11/1
  Delay47/1 -> Slice12/1
  gpio_set5/1 -> Delay23/1
  Constant8/1 -> gpio_set5/1
  gpio5/1 -> Scope5/1
  Slice14/1 -> gpio5/1, [gpioa5]
  Delay23/1 -> Slice14/1
  gpio_set4/1 -> Delay21/1
  Constant10/1 -> gpio_set4/1
  gpio4/1 -> Scope6/1
  Slice13/1 -> gpio4/1, [gpioa4]
  Delay21/1 -> Slice13/1
  Delay45/1 -> Slice15/1
  Delay46/1 -> Slice16/1
  Slice11/1 -> [wal0gpio], gpio6/1
  Slice12/1 -> [wal1gpio], gpio7/1
  gpio7/1 -> Scope1/1
  gpio6/1 -> Scope/1
  gpio/1 -> Scope7/1
  Slice16/1 -> gpio1/1, [wal3gpio]
  gpio1/1 -> Scope8/1
  [sync_gen] -> Counter2/1
  acc_sync_delay/1 -> Delay6/1
  Delay6/1 -> Slice20/1
  Slice20/1 -> Reinterpret/1
  Reinterpret/1 -> sync_delay_prog/2
  Delay64/1 -> Delay57/1
  Delay59/1 -> Delay58/1
  Delay61/1 -> Delay60/1
  Delay63/1 -> Delay62/1
  demodPhaseSwitch1/1 -> Delay3/1
  Constant15/1 -> demodPhaseSwitch1/1
  Delay3/1 -> Slice21/1
  Slice21/1 -> [demodPhaseSwitch]
  Constant16/1 -> phaseDelay2/1
  phaseDelay2/1 -> Delay31/1
  Delay31/1 -> [phaseDelay1]
  Delay57/1 -> Delay40/1
  Delay58/1 -> Delay42/1
  Delay60/1 -> Delay43/1
  Delay62/1 -> Delay44/1
  [Vsky_Add_Vload_LCP_Odd] -> Subsystem3/1(In1)
  [Vsky_Sub_Vload_LCP_Odd] -> Subsystem3/2(In2)
  [Vsky_Add_Vload_LCP_Even] -> Subsystem5/1(In1)
  [Vsky_Sub_Vload_LCP_Even] -> Subsystem5/2(In2)
  [Vsky_Add_Vload_RCP_Odd] -> Subsystem4/1(In1)
  [Vsky_Sub_Vload_RCP_Odd] -> Subsystem4/2(In2)
  [Vsky_Add_Vload_RCP_Even] -> Subsystem2/1(In1)
  [Vsky_Sub_Vload_RCP_Even] -> Subsystem2/2(In2)
  Subsystem3/1(Add) -> [Vsky_LCP_Odd]
  Subsystem3/2(Subtract) -> [VLoad_LCP_Odd]
  Subsystem5/1(Add) -> [Vsky_LCP_Even]
  Subsystem5/2(Subtract) -> [VLoad_LCP_Even]
  Subsystem4/1(Add) -> [Vsky_RCP_Odd]
  Subsystem4/2(Subtract) -> [VLoad_RCP_Odd]
  Subsystem2/1(Add) -> [Vsky_RCP_Even]
  Subsystem2/2(Subtract) -> [VLoad_RCP_Even]
  amp_EQ0/1(dout) -> [Vsky_Add_Vload_RCP_Even]
  amp_EQ1/1(dout) -> [Vsky_Add_Vload_RCP_Odd]
  amp_EQ2/1(dout) -> [Vsky_Sub_Vload_RCP_Even]
  amp_EQ3/1(dout) -> [Vsky_Sub_Vload_RCP_Odd]
  amp_EQ1/2(sync_out) -> [eq1_sync]
  amp_EQ0/2(sync_out) -> [eq_sync]
  amp_EQ2/2(sync_out) -> [eq2_sync]
  amp_EQ3/2(sync_out) -> [eq3_sync]
  amp_EQ4/2(sync_out) -> [eq4_sync]
  amp_EQ5/2(sync_out) -> [eq5_sync]
  amp_EQ6/2(sync_out) -> [eq6_sync]
  amp_EQ7/2(sync_out) -> [eq7_sync]
  amp_EQ6/1(dout) -> [Vsky_Sub_Vload_LCP_Even]
  amp_EQ7/1(dout) -> [Vsky_Sub_Vload_LCP_Odd]
  amp_EQ5/1(dout) -> [Vsky_Add_Vload_LCP_Odd]
  amp_EQ4/1(dout) -> [Vsky_Add_Vload_LCP_Even]
  [Vsky_RCP_Even] -> StokesDetector/2(RCP_Even)
  [Vsky_RCP_Odd] -> StokesDetector/3(RCP_Odd)
  [Vsky_LCP_Even] -> StokesDetector/4(LCP_Even)
  [Vsky_LCP_Odd] -> StokesDetector/5(LCP_Odd)
  [VLoad_RCP_Even] -> StokesDetector/6(RCP_Even_Load)
  [VLoad_RCP_Odd] -> StokesDetector/7(RCP_Odd_Load)
  [VLoad_LCP_Even] -> StokesDetector/8(LCP_Even_Load)
  [VLoad_LCP_Odd] -> StokesDetector/9(LCP_Odd_Load)
  StokesDetector/2(RCP_Even_Pow) -> Delay66/1
  StokesDetector/3(RCP_Odd_Pow) -> Delay51/1
  StokesDetector/4(LCP_Even_Pow) -> Delay53/1
  StokesDetector/5(LCP_Odd_Pow) -> Delay56/1
  StokesDetector/6(Q_Even) -> Delay64/1
  StokesDetector/7(Q_Odd) -> Delay59/1
  StokesDetector/8(U_Even) -> Delay61/1
  StokesDetector/9(U_Odd) -> Delay63/1
  Delay66/1 -> Delay35/1
  Delay51/1 -> Delay50/1
  Delay53/1 -> Delay52/1
  Delay56/1 -> Delay54/1
  Delay35/1 -> Delay36/1
  Delay50/1 -> Delay37/1
  Delay52/1 -> Delay38/1
  Delay54/1 -> Delay39/1
  Delay72/1 -> Delay32/1
  Delay67/1 -> Delay65/1
  Delay69/1 -> Delay68/1
  Delay71/1 -> Delay70/1
  Delay32/1 -> Delay33/1
  Delay65/1 -> Delay34/1
  Delay68/1 -> Delay48/1
  Delay70/1 -> Delay49/1
  StokesDetector/10(RCP_Even_Load_Pow) -> Delay72/1
  StokesDetector/11(RCP_Odd_Load_Pow) -> Delay67/1
  StokesDetector/12(LCP_Even_Load_Pow) -> Delay69/1
  StokesDetector/13(LCP_Odd_Load_Pow) -> Delay71/1
  Delay36/1 -> Subsystem1/2(Ch1)
  Delay37/1 -> Subsystem1/3(Ch2)
  Delay38/1 -> Subsystem1/4(Ch3)
  Delay39/1 -> Subsystem1/5(Ch4)
  Delay40/1 -> Subsystem1/6(Ch5)
  Delay42/1 -> Subsystem1/7(Ch6)
  Delay43/1 -> Subsystem1/8(Ch7)
  Delay44/1 -> Subsystem1/9(Ch8)
  Delay49/1 -> Subsystem1/13(Ch12)
  Delay48/1 -> Subsystem1/12(Ch11)
  Delay34/1 -> Subsystem1/11(Ch10)
  Delay33/1 -> Subsystem1/10(Ch9)
  sync_delay_prog/1 -> Subsystem1/1(sync)
  StokesDetector/1(sync_out) -> sync_cnt1/1, sync_delay_prog/1
  [eq_sync] -> Delay73/1
  Delay73/1 -> StokesDetector/1(sync_in)
  [acc_len] -> Subsystem1/14(acc_len)
  Delay74/1 -> bofMode/1
  Real6/1 -> Delay74/1
  bofMode/1 -> Terminator1/1
  Delay75/1 -> bofVersion/1
  Real7/1 -> Delay75/1
  bofVersion/1 -> Terminator2/1
  [adc0_lcp0] -> [adc0_lcp0demod]
  [adc0_lcp1] -> [adc0_lcp1demod]
  [adc0_lcp2] -> [adc0_lcp2demod]
  [adc0_lcp3] -> [adc0_lcp3demod]
  [adc0_lcp0a] -> [adc0_lcp0ademod]
  [adc0_lcp1a] -> [adc0_lcp1ademod]
  [adc0_lcp2a] -> [adc0_lcp2ademod]
  [adc0_lcp3a] -> [adc0_lcp3ademod]
  [adc0_rcp0] -> [adc0_rcp0demod]
  [adc0_rcp1] -> [adc0_rcp1demod]
  [adc0_rcp2] -> [adc0_rcp2demod]
  [adc0_rcp3] -> [adc0_rcp3demod]
  [adc0_rcp0a] -> [adc0_rcp0ademod]
  [adc0_rcp1a] -> [adc0_rcp1ademod]
  [adc0_rcp2a] -> [adc0_rcp2ademod]
  [adc0_rcp3a] -> [adc0_rcp3ademod]
  Real2/1 -> GPIOB_DIRECTION/1
  GPIOB_DIRECTION/1 -> Terminator4/1
  gpio10/1 -> Scope11/1
  gpio11/1 -> Scope12/1
  gpio13/1 -> Scope13/1
  gpio12/1 -> Scope14/1
  gpio15/1 -> Scope10/1
  gpio14/1 -> Scope9/1
  gpio8/1 -> Scope15/1
  gpio9/1 -> Scope16/1
  gpiob_set0/1 -> Delay79/1
  Constant14/1 -> gpiob_set0/1
  Slice17/1 -> gpio8/1, [gpiob0]
  Delay79/1 -> Slice17/1
  gpiob_set1/1 -> Delay80/1
  Constant17/1 -> gpiob_set1/1
  Delay80/1 -> Slice23/1
  Slice23/1 -> gpio9/1, [gpiob1]
  gpiob_set2/1 -> Delay55/1
  Constant11/1 -> gpiob_set2/1
  Delay55/1 -> Slice24/1
  Slice24/1 -> gpio10/1, [gpiob2]
  gpiob_set3/1 -> Delay76/1
  Constant12/1 -> gpiob_set3/1
  Delay76/1 -> Slice25/1
  Slice25/1 -> gpio11/1, [gpiob3]
  gpiob_set4/1 -> Delay77/1
  Constant13/1 -> gpiob_set4/1
  Delay77/1 -> Slice26/1
  Slice26/1 -> gpio12/1, [gpiob4]
  gpiob_set5/1 -> Delay78/1
  Constant19/1 -> gpiob_set5/1
  Delay78/1 -> Slice27/1
  Slice27/1 -> gpio13/1
  gpiob_set6/1 -> Delay81/1
  Constant20/1 -> gpiob_set6/1
  Delay81/1 -> Slice28/1
  Slice28/1 -> gpio14/1, [gpiob6]
  gpiob_set7/1 -> Delay82/1
  Constant21/1 -> gpiob_set7/1
  Delay82/1 -> Slice29/1
  Slice29/1 -> gpio15/1, [gpiob7]
  gpioMode/1 -> Delay83/1
  Constant22/1 -> gpioMode/1
  Delay83/1 -> Slice30/1
  gpio_set1/1 -> Delay85/1
  gpio_set2/1 -> Delay86/1
  gpio_set6/1 -> Delay87/1
  gpio_set7/1 -> Delay88/1
  Constant24/1 -> gpio_set1/1
  Constant23/1 -> gpio_set0/1
  Constant25/1 -> gpio_set2/1
  Constant26/1 -> gpio_set6/1
  Constant27/1 -> gpio_set7/1
  Slice30/1 -> [gpioMode]
  [gpioMode] -> Mux/1
  gpio_set0/1 -> Delay84/1
  Delay84/1 -> Slice31/1
  Delay85/1 -> Slice32/1
  Delay86/1 -> Slice33/1
  Delay87/1 -> Slice34/1
  Delay88/1 -> Slice35/1
  Slice15/1 -> gpio/1, [wal2gpio]
  Slice31/1 -> Mux/2
  [gpioMode] -> Mux1/1
  Slice32/1 -> Mux1/2
  [wal3] -> Mux1/3
  [wal2] -> Mux/3
  Mux/1 -> Delay45/1
  Mux1/1 -> Delay46/1
  [gpioMode] -> Mux2/1
  Slice33/1 -> Mux2/2
  Mux2/1 -> Delay20/1
  [gpioMode] -> Mux3/1
  Slice34/1 -> Mux3/2
  [wal0] -> Mux3/3
  Mux3/1 -> Delay41/1
  [gpioMode] -> Mux4/1
  Mux4/1 -> Delay47/1
  Delay89/1 -> Slice36/1
  Slice36/1 -> Mux2/3
  Counter2/1 -> Delay89/1
  Slice35/1 -> Mux4/2
  [wal1] -> Mux4/3
  Delay94/1 -> Concat/1
  Delay95/1 -> Concat/2
  Delay96/1 -> Concat/3
  Delay97/1 -> Concat/4
  Delay98/1 -> Concat/5
  Delay99/1 -> Concat/6
  Delay100/1 -> Concat/7
  Delay101/1 -> Concat/8
  Delay102/1 -> Concat/9
  [gpiob0] -> Delay94/1
  [gpiob1] -> Delay95/1
  [gpiob2] -> Delay96/1
  [gpiob3] -> Delay97/1
  [gpiob4] -> Delay98/1
  [gpiob6] -> Delay99/1
  [gpiob7] -> Delay100/1
  [gpioa3] -> Delay101/1
  [gpioa4] -> Delay102/1
  Delay93/1 -> statusReadout/1(reg_out)
  Concat/1 -> Delay93/1
  Relational/1 -> posedge1/1
  Slice8/1 -> Delay9/1
  Slice7/1 -> Delay8/1
  Delay9/1 -> sync/2
  sync_rst/1 -> Delay90/1
  Delay90/1 -> Slice7/1
  sync_en/1 -> Delay10/1
  Delay10/1 -> Slice8/1
  Constant7/1 -> sync_en/1
  posedge1/1 -> sync1/2, Logical4/2, Logical/2
  [sync_adc0] -> posedge6/1
  posedge6/1 -> sync1/1, Logical4/1, Logical/1
  Logical/1 -> [sync_gen]
  Delay8/1 -> Logical2/2
  Logical2/1 -> sync/1
  sync_max/1 -> Delay91/1
  Constant5/1 -> sync_max/1
  Delay91/1 -> Relational/2
  sync/1 -> Relational/1
  Delay7/1 -> no_PPS_cnt/1
  sync1/1 -> Delay7/1
  Logical4/1 -> Logical2/1

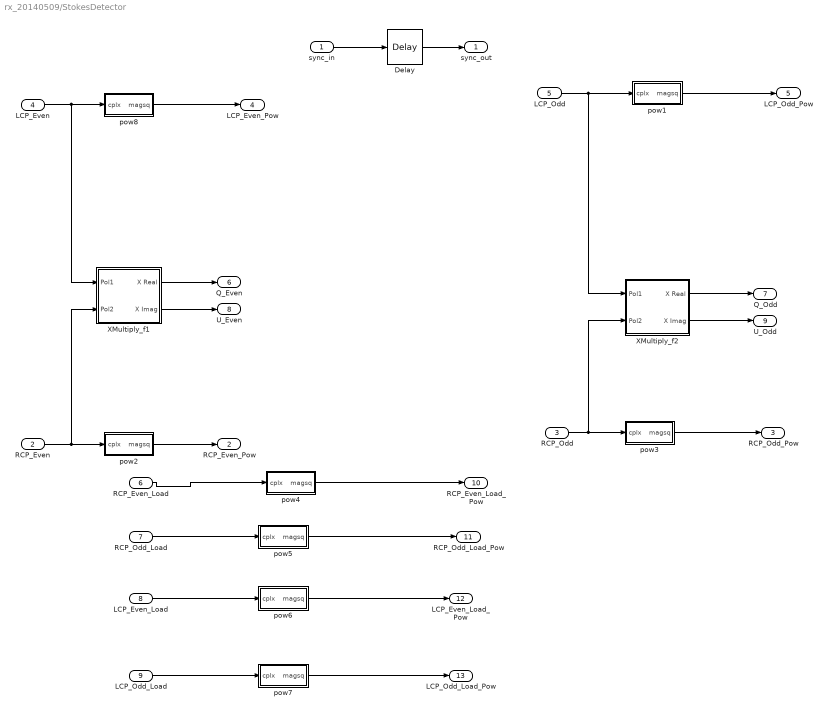
== system rx_20140509/StokesDetector ==
  sync_in : Inport
  RCP_Even : Inport  Port=2
  RCP_Odd : Inport  Port=3
  LCP_Even : Inport  Port=4
  LCP_Odd : Inport  Port=5
  RCP_Even_Load : Inport  Port=6
  RCP_Odd_Load : Inport  Port=7
  LCP_Even_Load : Inport  Port=8
  LCP_Odd_Load : Inport  Port=9
  Delay : xbsIndex_r4/Delay  rst=off  infoeditControl=Selection of Reset will increase slice count due to use of real FFs and instead of SRLs  en=off  latency=add_latency + mult_latency+3  dbl_ovrd=off  reg_retiming=on  block_type=delay
      settings: xl_area=[0, 0, 0, 0, 0, 0, 0]  block_version=10.1.2
  XMultiply_f1 : Subsystem
  XMultiply_f2 : Subsystem
  pow1 : Subsystem  AncestorBlock=gavrt_library/pow  mask{bit_width=18, add_latency=2, mult_latency=3}
      mask prompts: bit_width "Bit Width"; add_latency "Add Latency"; mult_latency "Mult Latency"
  pow2 : Subsystem  AncestorBlock=gavrt_library/pow  mask{bit_width=18, add_latency=2, mult_latency=3}
      mask prompts: bit_width "Bit Width"; add_latency "Add Latency"; mult_latency "Mult Latency"
  pow3 : Subsystem  AncestorBlock=gavrt_library/pow  mask{bit_width=18, add_latency=2, mult_latency=3}
      mask prompts: bit_width "Bit Width"; add_latency "Add Latency"; mult_latency "Mult Latency"
  pow4 : Subsystem  AncestorBlock=gavrt_library/pow  mask{bit_width=18, add_latency=2, mult_latency=3}
      mask prompts: bit_width "Bit Width"; add_latency "Add Latency"; mult_latency "Mult Latency"
  pow5 : Subsystem  AncestorBlock=gavrt_library/pow  mask{bit_width=18, add_latency=2, mult_latency=3}
      mask prompts: bit_width "Bit Width"; add_latency "Add Latency"; mult_latency "Mult Latency"
  pow6 : Subsystem  AncestorBlock=gavrt_library/pow  mask{bit_width=18, add_latency=2, mult_latency=3}
      mask prompts: bit_width "Bit Width"; add_latency "Add Latency"; mult_latency "Mult Latency"
  pow7 : Subsystem  AncestorBlock=gavrt_library/pow  mask{bit_width=18, add_latency=2, mult_latency=3}
      mask prompts: bit_width "Bit Width"; add_latency "Add Latency"; mult_latency "Mult Latency"
  pow8 : Subsystem  AncestorBlock=gavrt_library/pow  mask{bit_width=18, add_latency=2, mult_latency=3}
      mask prompts: bit_width "Bit Width"; add_latency "Add Latency"; mult_latency "Mult Latency"
  sync_out : Outport
  RCP_Even_Pow : Outport  Port=2
  RCP_Odd_Pow : Outport  Port=3
  LCP_Even_Pow : Outport  Port=4
  LCP_Odd_Pow : Outport  Port=5
  Q_Even : Outport  Port=6
  Q_Odd : Outport  Port=7
  U_Even : Outport  Port=8
  U_Odd : Outport  Port=9
  RCP_Even_Load_Pow : Outport  Port=10
  RCP_Odd_Load_Pow : Outport  Port=11
  LCP_Even_Load_Pow : Outport  Port=12
  LCP_Odd_Load_Pow : Outport  Port=13
  wires:
  Delay/1 -> sync_out/1
  sync_in/1 -> Delay/1
  XMultiply_f1/2(X Imag) -> U_Even/1
  XMultiply_f2/2(X Imag) -> U_Odd/1
  XMultiply_f1/1(X Real) -> Q_Even/1
  XMultiply_f2/1(X Real) -> Q_Odd/1
  pow8/1(magsq) -> LCP_Even_Pow/1
  LCP_Even/1 -> XMultiply_f1/1(Pol1), pow8/1(cplx)
  RCP_Odd/1 -> pow3/1(cplx), XMultiply_f2/2(Pol2)
  LCP_Odd/1 -> pow1/1(cplx), XMultiply_f2/1(Pol1)
  RCP_Even/1 -> XMultiply_f1/2(Pol2), pow2/1(cplx)
  pow2/1(magsq) -> RCP_Even_Pow/1
  pow3/1(magsq) -> RCP_Odd_Pow/1
  pow1/1(magsq) -> LCP_Odd_Pow/1
  LCP_Odd_Load/1 -> pow7/1(cplx)
  LCP_Even_Load/1 -> pow6/1(cplx)
  RCP_Odd_Load/1 -> pow5/1(cplx)
  RCP_Even_Load/1 -> pow4/1(cplx)
  pow7/1(magsq) -> LCP_Odd_Load_Pow/1
  pow6/1(magsq) -> LCP_Even_Load_Pow/1
  pow5/1(magsq) -> RCP_Odd_Load_Pow/1
  pow4/1(magsq) -> RCP_Even_Load_Pow/1
